simulink library "motion"  (Simulink 4.00)
undefined symbols (not defined in the file or in its folder): A6, Ac, Acd, ad, Aff, Aff0, Aff6, Ap, As, B6, Bc, Bcd, Bff, Bff0, Bff6, Bp, Bs, C6, Cc, Ccd, Cff, Cff0, Cff6, Cp, Cs, D6, Dc, dd, Ddd, Dff, Dff0, Dff6, Dp, Ds, jd, Ts, Tsettle
libraries: motion x5
(part 2 of 4)

== system motion/Feedforward Controllers/Feedforward ==
  In1 : Inport  Port=1
  4th order continuous : motion/Feedforward Controllers/4th order continuous  m1=20  m2=10  k1=10  k2=10  c=6e5  k12=500
  Out1 : Outport  Port=1
  wires:
  In1/1 -> 4th order continuous/1
  4th order continuous/1 -> Out1/1

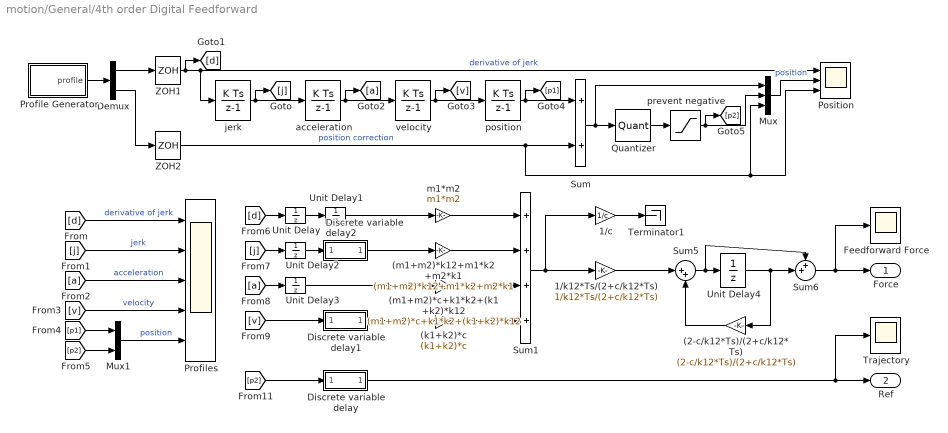
== system motion/General/4th order Digital Feedforward ==
  (2-c/k12*Ts)/(2+c/k12*Ts) : Gain  Orientation=left  Gain=(2-c/k12*Ts)/(2+c/k12*Ts)  Multiplication=Element-wise(K.*u)  SaturateOnIntegerOverflow=on
  (k1+k2)*c : Gain  Gain=(k1+k2)*c  Multiplication=Element-wise(K.*u)  SaturateOnIntegerOverflow=on
  (m1+m2)*c+k1*k2+(k1+k2)*k12 : Gain  Gain=(m1+m2)*c+k1*k2+(k1+k2)*k12  Multiplication=Element-wise(K.*u)  SaturateOnIntegerOverflow=on
  (m1+m2)*k12+m1*k2+m2*k1 : Gain  Gain=(m1+m2)*k12+m1*k2+m2*k1  Multiplication=Element-wise(K.*u)  SaturateOnIntegerOverflow=on
  1/c : Gain  Gain=1/c  Multiplication=Element-wise(K.*u)  SaturateOnIntegerOverflow=on
  1/k12*Ts/(2+c/k12*Ts) : Gain  Gain=1/k12*Ts/(2+c/k12*Ts)  Multiplication=Element-wise(K.*u)  SaturateOnIntegerOverflow=on
  Demux : Demux  Outputs=2  BusSelectionMode=off
  Discrete variable delay : Subsystem  mask{Ts=Ts, alpha=.5}
      mask prompts: Ts "Sample time"; alpha "Delay factor (between 0 and 1)"
      settings: RTWFcnNameOpts=Auto  RTWFileNameOpts=Auto
      mask Display: disp(sprintf('%3.1f*Ts',alpha))
  Discrete variable delay1 : Subsystem  mask{Ts=Ts, alpha=.5}
      mask prompts: Ts "Sample time"; alpha "Delay factor (between 0 and 1)"
      settings: RTWFcnNameOpts=Auto  RTWFileNameOpts=Auto
      mask Display: disp(sprintf('%3.1f*Ts',alpha))
  Discrete variable delay2 : Subsystem  mask{Ts=Ts, alpha=.5}
      mask prompts: Ts "Sample time"; alpha "Delay factor (between 0 and 1)"
      settings: RTWFcnNameOpts=Auto  RTWFileNameOpts=Auto
      mask Display: disp(sprintf('%3.1f*Ts',alpha))
  Feedforward Force : Scope
      settings: TimeRange=3  YMin=-150  YMax=200  SaveToWorkspace=off  SaveName=ScopeData  LimitDataPoints=on  MaxDataPoints=50000
  Mux : Mux  Inputs=3
  Mux1 : Mux  Inputs=2
  Position : Scope  NumInputPorts=3
      settings: TimeRange=3  YMin=-1000~-0.5~-0.0004  YMax=1000~1~0  SaveToWorkspace=off  SaveName=ScopeData2  LimitDataPoints=on  MaxDataPoints=50000
  Profile Generator : Subsystem  BlockChoice=dJerk with error correction
      link override dJerk with error correction: t0=t0  x=x  v=v  a=a  j=j  d=d  Ts=Ts  r=r  s=s
      settings: AttributesFormatString=%<BlockChoice>  TemplateBlock=motion/Profile Generators/Profile Generator  MemberBlocks=Acceleration,Derivative of Jerk,Jerk,dJerk with error correction  RTWFcnNameOpts=Auto  RTWFileNameOpts=Auto
  Profiles : Scope  NumInputPorts=5
      settings: TimeRange=3  YMin=-1000~-50~-5~-7.49453e-017~0  YMax=1000~50~5~1~1  SaveToWorkspace=off  SaveName=ScopeData4  LimitDataPoints=on  MaxDataPoints=50000
  Quantizer : Quantizer  QuantizationInterval=r  LinearizeAsGain=on
  Sum : Sum  Inputs=++  SaturateOnIntegerOverflow=on
  Sum1 : Sum  Inputs=++++  SaturateOnIntegerOverflow=on
  Sum5 : Sum  Inputs=|++  SaturateOnIntegerOverflow=on
  Sum6 : Sum  Inputs=++|  SaturateOnIntegerOverflow=on
  Terminator1 : Terminator
  Trajectory : Scope
      settings: TimeRange=3  YMin=0  YMax=1  SaveToWorkspace=off  SaveName=ScopeData7  LimitDataPoints=on  MaxDataPoints=50000
  Unit Delay{,1..4} (5 alike) : UnitDelay  X0=0  SampleTime=Ts
  ZOH1 : ZeroOrderHold  SampleTime=Ts
  ZOH2 : ZeroOrderHold  SampleTime=Ts
  acceleration : DiscreteIntegrator  IntegratorMethod=ForwardEuler  ExternalReset=none  InitialConditionSource=internal  InitialCondition=0  LimitOutput=off  UpperSaturationLimit=inf  LowerSaturationLimit=-inf  ShowSaturationPort=off  ShowStatePort=off  SampleTime=Ts
  jerk : DiscreteIntegrator  IntegratorMethod=ForwardEuler  ExternalReset=none  InitialConditionSource=internal  InitialCondition=0  LimitOutput=off  UpperSaturationLimit=inf  LowerSaturationLimit=-inf  ShowSaturationPort=off  ShowStatePort=off  SampleTime=Ts
  m1*m2 : Gain  Gain=m1*m2  Multiplication=Element-wise(K.*u)  SaturateOnIntegerOverflow=on
  position : DiscreteIntegrator  IntegratorMethod=ForwardEuler  ExternalReset=none  InitialConditionSource=internal  InitialCondition=0  LimitOutput=off  UpperSaturationLimit=inf  LowerSaturationLimit=-inf  ShowSaturationPort=off  ShowStatePort=off  SampleTime=Ts
  "prevent negative " : Saturate  UpperLimit=inf  LowerLimit=0  LinearizeAsGain=on
  velocity : DiscreteIntegrator  IntegratorMethod=ForwardEuler  ExternalReset=none  InitialConditionSource=internal  InitialCondition=0  LimitOutput=off  UpperSaturationLimit=inf  LowerSaturationLimit=-inf  ShowSaturationPort=off  ShowStatePort=off  SampleTime=Ts
  Force : Outport  Port=1
  Ref : Outport  Port=2
  wires:
  m1*m2/1 -> Sum1/1
  Profile Generator/1(profile) -> Demux/1
  (m1+m2)*k12+m1*k2+m2*k1/1 -> Sum1/2
  1/c/1 -> Terminator1/1
  Sum6/1 -> Force/1, Feedforward Force/1
  (2-c/k12*Ts)/(2+c/k12*Ts)/1 -> Sum5/2
  Unit Delay4/1 -> Sum6/2, (2-c/k12*Ts)/(2+c/k12*Ts)/1
  Sum5/1 -> Sum6/1, Unit Delay4/1
  1/k12*Ts/(2+c/k12*Ts)/1 -> Sum5/1
  Discrete variable delay2/1(Out1) -> (m1+m2)*k12+m1*k2+m2*k1/1
  Discrete variable delay1/1(Out1) -> (k1+k2)*c/1
  Unit Delay3/1 -> (m1+m2)*c+k1*k2+(k1+k2)*k12/1
  Unit Delay2/1 -> Discrete variable delay2/1(In1)
  Unit Delay1/1 -> m1*m2/1
  Unit Delay/1 -> Unit Delay1/1
  "prevent negative "/1 -> [p2], Mux/2
  Discrete variable delay/1(Out1) -> Ref/1, Trajectory/1
  [p2] -> Discrete variable delay/1(In1)
  Sum1/1 -> 1/k12*Ts/(2+c/k12*Ts)/1, 1/c/1
  (k1+k2)*c/1 -> Sum1/4
  (m1+m2)*c+k1*k2+(k1+k2)*k12/1 -> Sum1/3
  [v] -> Discrete variable delay1/1(In1)
  [a] -> Unit Delay3/1
  [j] -> Unit Delay2/1
  [d] -> Unit Delay/1
  Mux1/1 -> Profiles/5  "position"
  [v] -> Profiles/4  "velocity"
  [a] -> Profiles/3  "acceleration"
  [j] -> Profiles/2  "jerk"
  [d] -> Profiles/1  "derivative of jerk"
  [p2] -> Mux1/2
  [p1] -> Mux1/1
  ZOH2/1 -> Position/3, Mux/3, Sum/2  "position correction"
  position/1 -> [p1], Sum/1
  Mux/1 -> Position/2  "position"
  Sum/1 -> Mux/1, Quantizer/1
  Quantizer/1 -> "prevent negative "/1
  Demux/2 -> ZOH2/1
  ZOH1/1 -> [d], Position/1, jerk/1  "derivative of jerk"
  velocity/1 -> [v], position/1
  acceleration/1 -> [a], velocity/1
  jerk/1 -> [j], acceleration/1
  Demux/1 -> ZOH1/1

== system motion/General/open example ==
  note: Run makeplant

== system motion/General/open example1 ==
  note: Run makeplant

== system motion/General/open example2 ==
  note: Run makeplant

== system motion/General/run makeplant ==
  note: Run makeplant

== system motion/Motion Systems1/Motion System ==
  In1 : Inport  Port=1
  2nd order : StateSpace  A=As  B=Bs  C=Cs  D=Ds  X0=0  Realization=auto  AbsoluteTolerance=auto
  Out1 : Outport  Port=1
  wires:
  In1/1 -> 2nd order/1
  2nd order/1 -> Out1/1

== system motion/Motion Systems1/Parametrized 4th order ==
  In1 : Inport  Port=1
  4th order plant1 : StateSpace  A=Ap  B=Bp  C=Cp  D=Dp  X0=0  Realization=auto  AbsoluteTolerance=auto
  Out1 : Outport  Port=1
  wires:
  4th order plant1/1 -> Out1/1
  In1/1 -> 4th order plant1/1

== system motion/Profile Generators/Acceleration ==
  Sum : Sum  Inputs=4  SaturateOnIntegerOverflow=on
  t0 : Step  Time=t0  Before=0  After=ad(1)  SampleTime=0
  t1 : Step  Time=t0+t(1)  Before=0  After=-ad(1)  SampleTime=0
  t2 : Step  Time=t0+t(1)+t(2)  Before=0  After=-ad(1)  SampleTime=0
  t3 : Step  Time=t0+2*t(1)+t(2)  Before=0  After=ad(1)  SampleTime=0
  profile : Outport  Port=1
  wires:
  t0/1 -> Sum/1
  t1/1 -> Sum/2
  t2/1 -> Sum/3
  t3/1 -> Sum/4
  Sum/1 -> profile/1

== system motion/Profile Generators/Derivative of Jerk ==
  Sum : Sum  Inputs=16  SaturateOnIntegerOverflow=on
  t0 : Step  Time=t0  Before=0  After=dd(1)  SampleTime=0
  t1 : Step  Time=t0+t(1)  Before=0  After=-dd(1)  SampleTime=0
  t10 : Step  Time=t0+5*t(1)+3*t(2)+t(3)+t(4)  Before=0  After=dd(1)  SampleTime=0
  t11 : Step  Time=t0+6*t(1)+3*t(2)+t(3)+t(4)  Before=0  After=-dd(1)  SampleTime=0
  t12 : Step  Time=t0+6*t(1)+3*t(2)+2*t(3)+t(4)  Before=0  After=dd(1)  SampleTime=0
  t13 : Step  Time=t0+7*t(1)+3*t(2)+2*t(3)+t(4)  Before=0  After=-dd(1)  SampleTime=0
  t14 : Step  Time=t0+7*t(1)+4*t(2)+2*t(3)+t(4)  Before=0  After=-dd(1)  SampleTime=0
  t15 : Step  Time=t0+8*t(1)+4*t(2)+2*t(3)+t(4)  Before=0  After=dd(1)  SampleTime=0
  t2 : Step  Time=t0+t(1)+t(2)  Before=0  After=-dd(1)  SampleTime=0
  t3 : Step  Time=t0+2*t(1)+t(2)  Before=0  After=dd(1)  SampleTime=0
  t4 : Step  Time=t0+2*t(1)+t(2)+t(3)  Before=0  After=-dd(1)  SampleTime=0
  t5 : Step  Time=t0+3*t(1)+t(2)+t(3)  Before=0  After=dd(1)  SampleTime=0
  t6 : Step  Time=t0+3*t(1)+2*t(2)+t(3)  Before=0  After=dd(1)  SampleTime=0
  t7 : Step  Time=t0+4*t(1)+2*t(2)+t(3)  Before=0  After=-dd(1)  SampleTime=0
  t8 : Step  Time=t0+4*t(1)+2*t(2)+t(3)+t(4)  Before=0  After=-dd(1)  SampleTime=0
  t9 : Step  Time=t0+5*t(1)+2*t(2)+t(3)+t(4)  Before=0  After=dd(1)  SampleTime=0
  profile : Outport  Port=1
  wires:
  t0/1 -> Sum/1
  t1/1 -> Sum/2
  t2/1 -> Sum/3
  t3/1 -> Sum/4
  t4/1 -> Sum/5
  t5/1 -> Sum/6
  t6/1 -> Sum/7
  t7/1 -> Sum/8
  t8/1 -> Sum/9
  t9/1 -> Sum/10
  t10/1 -> Sum/11
  t11/1 -> Sum/12
  t12/1 -> Sum/13
  t13/1 -> Sum/14
  t14/1 -> Sum/15
  t15/1 -> Sum/16
  Sum/1 -> profile/1

== system motion/Profile Generators/Jerk ==
  Sum : Sum  Inputs=8  SaturateOnIntegerOverflow=on
  t0 : Step  Time=t0  Before=0  After=jd(1)  SampleTime=0
  t1 : Step  Time=t0+t(1)  Before=0  After=-jd(1)  SampleTime=0
  t2 : Step  Time=t0+t(1)+t(2)  Before=0  After=-jd(1)  SampleTime=0
  t3 : Step  Time=t0+2*t(1)+t(2)  Before=0  After=jd(1)  SampleTime=0
  t4 : Step  Time=t0+2*t(1)+t(2)+t(3)  Before=0  After=-jd(1)  SampleTime=0
  t5 : Step  Time=t0+3*t(1)+t(2)+t(3)  Before=0  After=jd(1)  SampleTime=0
  t6 : Step  Time=t0+3*t(1)+2*t(2)+t(3)  Before=0  After=jd(1)  SampleTime=0
  t7 : Step  Time=t0+4*t(1)+2*t(2)+t(3)  Before=0  After=-jd(1)  SampleTime=0
  profile : Outport  Port=1
  wires:
  Sum/1 -> profile/1
  t7/1 -> Sum/8
  t6/1 -> Sum/7
  t5/1 -> Sum/6
  t4/1 -> Sum/5
  t3/1 -> Sum/4
  t2/1 -> Sum/3
  t1/1 -> Sum/2
  t0/1 -> Sum/1

== system motion/Profile Generators/Profile Generator ==
  Acceleration : motion/Profile Generators/Acceleration  t0=.3  x=1  v=1  a=5  Ts=0
  profile : Outport  Port=1
  wires:
  Acceleration/1 -> profile/1

== system motion/Profile Generators/dJerk with error correction ==
  Clock : Clock
      settings: DisplayTime=off  Decimation=10
  Correction at start of trajectory : Lookup  InputValues="[ -1 t0 t0+abs(dd(3))*Ts  2*(t0+8*t(1)+4*t(2)+2*t(3)+t(4)) ]"  OutputValues=[ 0 0 [1 1]*dd(3)*r]
  Correction during entire trajectory : Lookup  InputValues="[ -1 t0  t0+8*t(1)+4*t(2)+2*t(3)+t(4)  2*(t0+8*t(1)+4*t(2)+2*t(3)+t(4)) ]"  OutputValues=[0 0 [1 1]*dd(2)*r]
  Mux : Mux  Inputs=2
  Sum : Sum  Inputs=16  SaturateOnIntegerOverflow=on
  Sum1 : Sum  Inputs=|++  SaturateOnIntegerOverflow=on
  t0 : Step  Time=t0  Before=0  After=dd(1)  SampleTime=0
  t1 : Step  Time=t0+t(1)  Before=0  After=-dd(1)  SampleTime=0
  t10 : Step  Time=t0+5*t(1)+3*t(2)+t(3)+t(4)  Before=0  After=dd(1)  SampleTime=0
  t11 : Step  Time=t0+6*t(1)+3*t(2)+t(3)+t(4)  Before=0  After=-dd(1)  SampleTime=0
  t12 : Step  Time=t0+6*t(1)+3*t(2)+2*t(3)+t(4)  Before=0  After=dd(1)  SampleTime=0
  t13 : Step  Time=t0+7*t(1)+3*t(2)+2*t(3)+t(4)  Before=0  After=-dd(1)  SampleTime=0
  t14 : Step  Time=t0+7*t(1)+4*t(2)+2*t(3)+t(4)  Before=0  After=-dd(1)  SampleTime=0
  t15 : Step  Time=t0+8*t(1)+4*t(2)+2*t(3)+t(4)  Before=0  After=dd(1)  SampleTime=0
  t2 : Step  Time=t0+t(1)+t(2)  Before=0  After=-dd(1)  SampleTime=0
  t3 : Step  Time=t0+2*t(1)+t(2)  Before=0  After=dd(1)  SampleTime=0
  t4 : Step  Time=t0+2*t(1)+t(2)+t(3)  Before=0  After=-dd(1)  SampleTime=0
  t5 : Step  Time=t0+3*t(1)+t(2)+t(3)  Before=0  After=dd(1)  SampleTime=0
  t6 : Step  Time=t0+3*t(1)+2*t(2)+t(3)  Before=0  After=dd(1)  SampleTime=0
  t7 : Step  Time=t0+4*t(1)+2*t(2)+t(3)  Before=0  After=-dd(1)  SampleTime=0
  t8 : Step  Time=t0+4*t(1)+2*t(2)+t(3)+t(4)  Before=0  After=-dd(1)  SampleTime=0
  t9 : Step  Time=t0+5*t(1)+2*t(2)+t(3)+t(4)  Before=0  After=dd(1)  SampleTime=0
  profile : Outport  Port=1
  wires:
  Sum/1 -> Mux/1
  Mux/1 -> profile/1
  t0/1 -> Sum/1
  t1/1 -> Sum/2
  t2/1 -> Sum/3
  t3/1 -> Sum/4
  t4/1 -> Sum/5
  t5/1 -> Sum/6
  t6/1 -> Sum/7
  t7/1 -> Sum/8
  t8/1 -> Sum/9
  t9/1 -> Sum/10
  t10/1 -> Sum/11
  t11/1 -> Sum/12
  t12/1 -> Sum/13
  t13/1 -> Sum/14
  t14/1 -> Sum/15
  t15/1 -> Sum/16
  Clock/1 -> Correction during entire trajectory/1, Correction at start of trajectory/1
  Correction at start of trajectory/1 -> Sum1/2
  Sum1/1 -> Mux/2
  Correction during entire trajectory/1 -> Sum1/1

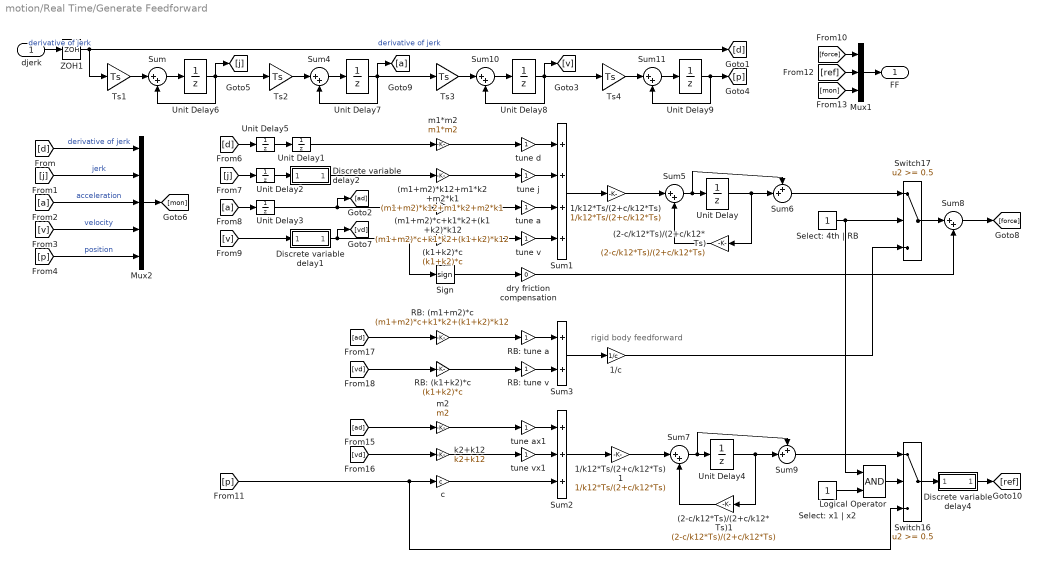
== system motion/Real Time/Generate Feedforward ==
  note: rigid body feedforward
  djerk : Inport  Port=1
  (2-c/k12*Ts)/(2+c/k12*Ts) : Gain  Orientation=left  Gain=(2-c/k12*Ts)/(2+c/k12*Ts)  Multiplication=Element-wise(K.*u)  SaturateOnIntegerOverflow=on
  (2-c/k12*Ts)/(2+c/k12*Ts)1 : Gain  Orientation=left  Gain=(2-c/k12*Ts)/(2+c/k12*Ts)  Multiplication=Element-wise(K.*u)  SaturateOnIntegerOverflow=on
  (k1+k2)*c : Gain  Gain=(k1+k2)*c  Multiplication=Element-wise(K.*u)  SaturateOnIntegerOverflow=on
  (m1+m2)*c+k1*k2+(k1+k2)*k12 : Gain  Gain=(m1+m2)*c+k1*k2+(k1+k2)*k12  Multiplication=Element-wise(K.*u)  SaturateOnIntegerOverflow=on
  (m1+m2)*k12+m1*k2+m2*k1 : Gain  Gain=(m1+m2)*k12+m1*k2+m2*k1  Multiplication=Element-wise(K.*u)  SaturateOnIntegerOverflow=on
  1/c : Gain  Gain=1/c  Multiplication=Element-wise(K.*u)  SaturateOnIntegerOverflow=on
  1/k12*Ts/(2+c/k12*Ts) : Gain  Gain=1/k12*Ts/(2+c/k12*Ts)  Multiplication=Element-wise(K.*u)  SaturateOnIntegerOverflow=on
  1/k12*Ts/(2+c/k12*Ts)1 : Gain  Gain=1/k12*Ts/(2+c/k12*Ts)  Multiplication=Element-wise(K.*u)  SaturateOnIntegerOverflow=on
  Discrete variable delay1 : Subsystem  mask{Ts=Ts, alpha=.5}
      mask prompts: Ts "Sample time"; alpha "Delay factor (between 0 and 1)"
      settings: RTWFcnNameOpts=Auto  RTWFileNameOpts=Auto
      mask Display: disp(sprintf('%3.1f*Ts',alpha))
  Discrete variable delay2 : Subsystem  mask{Ts=Ts, alpha=.5}
      mask prompts: Ts "Sample time"; alpha "Delay factor (between 0 and 1)"
      settings: RTWFcnNameOpts=Auto  RTWFileNameOpts=Auto
      mask Display: disp(sprintf('%3.1f*Ts',alpha))
  Discrete variable delay4 : Subsystem  mask{Ts=Ts, alpha=.5}
      mask prompts: Ts "Sample time"; alpha "Delay factor (between 0 and 1)"
      settings: RTWFcnNameOpts=Auto  RTWFileNameOpts=Auto
      mask Display: disp(sprintf('%3.1f*Ts',alpha))
  Logical Operator : Logic  Operator=AND  Inputs=2
  Mux1 : Mux  Inputs=3
  Mux2 : Mux  Inputs=5
  RB: (k1+k2)*c : Gain  Gain=(k1+k2)*c  Multiplication=Element-wise(K.*u)  SaturateOnIntegerOverflow=on
  RB: (m1+m2)*c : Gain  Gain=(m1+m2)*c+k1*k2+(k1+k2)*k12  Multiplication=Element-wise(K.*u)  SaturateOnIntegerOverflow=on
  RB: tune a : Gain  Gain=1  Multiplication=Element-wise(K.*u)  SaturateOnIntegerOverflow=on
  RB: tune v : Gain  Gain=1  Multiplication=Element-wise(K.*u)  SaturateOnIntegerOverflow=on
  Select: 4th | RB : Constant  Value=1
  Select: x1 | x2 : Constant  Value=1
  Sign : Signum
  Sum{,4..5,7..8,10..11} (7 alike) : Sum  Inputs=|++  SaturateOnIntegerOverflow=on
  Sum1 : Sum  Inputs=++++  SaturateOnIntegerOverflow=on
  Sum2 : Sum  Inputs=+++  SaturateOnIntegerOverflow=on
  Sum3 : Sum  Inputs=++  SaturateOnIntegerOverflow=on
  Sum6 : Sum  Inputs=++|  SaturateOnIntegerOverflow=on
  Sum9 : Sum  Inputs=++|  SaturateOnIntegerOverflow=on
  Switch16 : Switch  Threshold=0.5
  Switch17 : Switch  Threshold=0.5
  Ts{1..4} (4 alike) : Gain  Gain=Ts  Multiplication=Element-wise(K.*u)  SaturateOnIntegerOverflow=on
  Unit Delay{,1..9} (10 alike) : UnitDelay  X0=0  SampleTime=Ts
  ZOH1 : ZeroOrderHold  SampleTime=Ts
  c : Gain  Gain=c  Multiplication=Element-wise(K.*u)  SaturateOnIntegerOverflow=on
  dry friction compensation : Gain  Gain=0  Multiplication=Element-wise(K.*u)  SaturateOnIntegerOverflow=on
  k2+k12 : Gain  Gain=k2+k12  Multiplication=Element-wise(K.*u)  SaturateOnIntegerOverflow=on
  m1*m2 : Gain  Gain=m1*m2  Multiplication=Element-wise(K.*u)  SaturateOnIntegerOverflow=on
  m2 : Gain  Gain=m2  Multiplication=Element-wise(K.*u)  SaturateOnIntegerOverflow=on
  tune a : Gain  Gain=1  Multiplication=Element-wise(K.*u)  SaturateOnIntegerOverflow=on
  tune ax1 : Gain  Gain=1  Multiplication=Element-wise(K.*u)  SaturateOnIntegerOverflow=on
  tune d : Gain  Gain=1  Multiplication=Element-wise(K.*u)  SaturateOnIntegerOverflow=on
  tune j : Gain  Gain=1  Multiplication=Element-wise(K.*u)  SaturateOnIntegerOverflow=on
  tune v : Gain  Gain=1  Multiplication=Element-wise(K.*u)  SaturateOnIntegerOverflow=on
  tune vx1 : Gain  Gain=1  Multiplication=Element-wise(K.*u)  SaturateOnIntegerOverflow=on
  FF : Outport  Port=1
  wires:
  Sum11/1 -> Unit Delay9/1
  Ts4/1 -> Sum11/1
  Unit Delay9/1 -> [p], Sum11/2
  Sum10/1 -> Unit Delay8/1
  Ts3/1 -> Sum10/1
  Unit Delay8/1 -> Ts4/1, [v], Sum10/2
  Sum4/1 -> Unit Delay7/1
  Ts2/1 -> Sum4/1
  Unit Delay7/1 -> Ts3/1, [a], Sum4/2
  Sum/1 -> Unit Delay6/1
  Ts1/1 -> Sum/1
  Unit Delay6/1 -> Ts2/1, [j], Sum/2
  c/1 -> Sum2/3
  Select: 4th | RB/1 -> Logical Operator/1, Switch17/2
  Sum9/1 -> Switch16/1
  1/c/1 -> Switch17/3
  dry friction compensation/1 -> Sum8/2
  Logical Operator/1 -> Switch16/2
  Select: x1 | x2/1 -> Logical Operator/2
  Discrete variable delay4/1(Out1) -> [ref]
  Switch16/1 -> Discrete variable delay4/1(In1)
  Sum8/1 -> [force]
  Switch17/1 -> Sum8/1
  Sum6/1 -> Switch17/1
  Unit Delay4/1 -> Sum9/2, (2-c/k12*Ts)/(2+c/k12*Ts)1/1
  Sum7/1 -> Sum9/1, Unit Delay4/1
  1/k12*Ts/(2+c/k12*Ts)1/1 -> Sum7/1
  Sum2/1 -> 1/k12*Ts/(2+c/k12*Ts)1/1
  (2-c/k12*Ts)/(2+c/k12*Ts)1/1 -> Sum7/2
  [vd] -> k2+k12/1
  [ad] -> m2/1
  [p] -> c/1, Switch16/3
  m2/1 -> tune ax1/1
  tune ax1/1 -> Sum2/1
  k2+k12/1 -> tune vx1/1
  tune vx1/1 -> Sum2/2
  [ad] -> RB: (m1+m2)*c/1
  [vd] -> RB: (k1+k2)*c/1
  RB: (m1+m2)*c/1 -> RB: tune a/1
  RB: tune a/1 -> Sum3/1
  RB: (k1+k2)*c/1 -> RB: tune v/1
  RB: tune v/1 -> Sum3/2
  Sum3/1 -> 1/c/1
  [force] -> Mux1/1
  [ref] -> Mux1/2
  [mon] -> Mux1/3
  Mux1/1 -> FF/1
  Unit Delay3/1 -> [ad], (m1+m2)*c+k1*k2+(k1+k2)*k12/1
  Discrete variable delay2/1(Out1) -> (m1+m2)*k12+m1*k2+m2*k1/1
  Unit Delay1/1 -> m1*m2/1
  m1*m2/1 -> tune d/1
  tune d/1 -> Sum1/1
  (m1+m2)*k12+m1*k2+m2*k1/1 -> tune j/1
  tune j/1 -> Sum1/2
  (m1+m2)*c+k1*k2+(k1+k2)*k12/1 -> tune a/1
  tune a/1 -> Sum1/3
  (k1+k2)*c/1 -> tune v/1
  tune v/1 -> Sum1/4
  Unit Delay/1 -> Sum6/2, (2-c/k12*Ts)/(2+c/k12*Ts)/1
  Sum5/1 -> Sum6/1, Unit Delay/1
  1/k12*Ts/(2+c/k12*Ts)/1 -> Sum5/1
  Sum1/1 -> 1/k12*Ts/(2+c/k12*Ts)/1
  (2-c/k12*Ts)/(2+c/k12*Ts)/1 -> Sum5/2
  Sign/1 -> dry friction compensation/1
  djerk/1 -> ZOH1/1  "derivative of jerk"
  Unit Delay2/1 -> Discrete variable delay2/1(In1)
  Unit Delay5/1 -> Unit Delay1/1
  [v] -> Discrete variable delay1/1(In1)
  [a] -> Unit Delay3/1
  [j] -> Unit Delay2/1
  [d] -> Unit Delay5/1
  [v] -> Mux2/4  "velocity"
  [a] -> Mux2/3  "acceleration"
  [j] -> Mux2/2  "jerk"
  [d] -> Mux2/1  "derivative of jerk"
  [p] -> Mux2/5  "position"
  Mux2/1 -> [mon]
  ZOH1/1 -> Ts1/1, [d]  "derivative of jerk"
  Discrete variable delay1/1(Out1) -> [vd], (k1+k2)*c/1, Sign/1

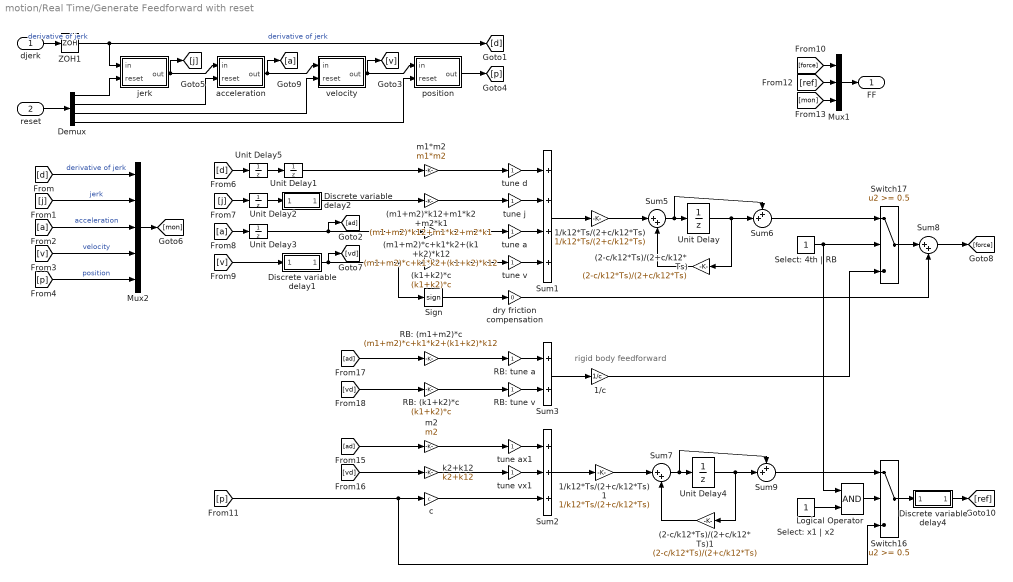
== system motion/Real Time/Generate Feedforward with reset ==
  note: rigid body feedforward
  djerk : Inport  Port=1
  reset : Inport  Port=2
  (2-c/k12*Ts)/(2+c/k12*Ts) : Gain  Orientation=left  Gain=(2-c/k12*Ts)/(2+c/k12*Ts)  Multiplication=Element-wise(K.*u)  SaturateOnIntegerOverflow=on
  (2-c/k12*Ts)/(2+c/k12*Ts)1 : Gain  Orientation=left  Gain=(2-c/k12*Ts)/(2+c/k12*Ts)  Multiplication=Element-wise(K.*u)  SaturateOnIntegerOverflow=on
  (k1+k2)*c : Gain  Gain=(k1+k2)*c  Multiplication=Element-wise(K.*u)  SaturateOnIntegerOverflow=on
  (m1+m2)*c+k1*k2+(k1+k2)*k12 : Gain  Gain=(m1+m2)*c+k1*k2+(k1+k2)*k12  Multiplication=Element-wise(K.*u)  SaturateOnIntegerOverflow=on
  (m1+m2)*k12+m1*k2+m2*k1 : Gain  Gain=(m1+m2)*k12+m1*k2+m2*k1  Multiplication=Element-wise(K.*u)  SaturateOnIntegerOverflow=on
  1/c : Gain  Gain=1/c  Multiplication=Element-wise(K.*u)  SaturateOnIntegerOverflow=on
  1/k12*Ts/(2+c/k12*Ts) : Gain  Gain=1/k12*Ts/(2+c/k12*Ts)  Multiplication=Element-wise(K.*u)  SaturateOnIntegerOverflow=on
  1/k12*Ts/(2+c/k12*Ts)1 : Gain  Gain=1/k12*Ts/(2+c/k12*Ts)  Multiplication=Element-wise(K.*u)  SaturateOnIntegerOverflow=on
  Demux : Demux  Outputs=4  BusSelectionMode=off
  Discrete variable delay1 : Subsystem  mask{Ts=Ts, alpha=.5}
      mask prompts: Ts "Sample time"; alpha "Delay factor (between 0 and 1)"
      settings: RTWFcnNameOpts=Auto  RTWFileNameOpts=Auto
      mask Display: disp(sprintf('%3.1f*Ts',alpha))
  Discrete variable delay2 : Subsystem  mask{Ts=Ts, alpha=.5}
      mask prompts: Ts "Sample time"; alpha "Delay factor (between 0 and 1)"
      settings: RTWFcnNameOpts=Auto  RTWFileNameOpts=Auto
      mask Display: disp(sprintf('%3.1f*Ts',alpha))
  Discrete variable delay4 : Subsystem  mask{Ts=Ts, alpha=.5}
      mask prompts: Ts "Sample time"; alpha "Delay factor (between 0 and 1)"
      settings: RTWFcnNameOpts=Auto  RTWFileNameOpts=Auto
      mask Display: disp(sprintf('%3.1f*Ts',alpha))
  Logical Operator : Logic  Operator=AND  Inputs=2
  Mux1 : Mux  Inputs=3
  Mux2 : Mux  Inputs=5
  RB: (k1+k2)*c : Gain  Gain=(k1+k2)*c  Multiplication=Element-wise(K.*u)  SaturateOnIntegerOverflow=on
  RB: (m1+m2)*c : Gain  Gain=(m1+m2)*c+k1*k2+(k1+k2)*k12  Multiplication=Element-wise(K.*u)  SaturateOnIntegerOverflow=on
  RB: tune a : Gain  Gain=1  Multiplication=Element-wise(K.*u)  SaturateOnIntegerOverflow=on
  RB: tune v : Gain  Gain=1  Multiplication=Element-wise(K.*u)  SaturateOnIntegerOverflow=on
  Select: 4th | RB : Constant  Value=1
  Select: x1 | x2 : Constant  Value=1
  Sign : Signum
  Sum1 : Sum  Inputs=++++  SaturateOnIntegerOverflow=on
  Sum2 : Sum  Inputs=+++  SaturateOnIntegerOverflow=on
  Sum3 : Sum  Inputs=++  SaturateOnIntegerOverflow=on
  Sum5 : Sum  Inputs=|++  SaturateOnIntegerOverflow=on
  Sum6 : Sum  Inputs=++|  SaturateOnIntegerOverflow=on
  Sum7 : Sum  Inputs=|++  SaturateOnIntegerOverflow=on
  Sum8 : Sum  Inputs=|++  SaturateOnIntegerOverflow=on
  Sum9 : Sum  Inputs=++|  SaturateOnIntegerOverflow=on
  Switch16 : Switch  Threshold=0.5
  Switch17 : Switch  Threshold=0.5
  Unit Delay{,1..5} (6 alike) : UnitDelay  X0=0  SampleTime=Ts
  ZOH1 : ZeroOrderHold  SampleTime=Ts
  acceleration : Subsystem
      settings: RTWFcnNameOpts=Auto  RTWFileNameOpts=Auto
  c : Gain  Gain=c  Multiplication=Element-wise(K.*u)  SaturateOnIntegerOverflow=on
  dry friction compensation : Gain  Gain=0  Multiplication=Element-wise(K.*u)  SaturateOnIntegerOverflow=on
  jerk : Subsystem
      settings: RTWFcnNameOpts=Auto  RTWFileNameOpts=Auto
  k2+k12 : Gain  Gain=k2+k12  Multiplication=Element-wise(K.*u)  SaturateOnIntegerOverflow=on
  m1*m2 : Gain  Gain=m1*m2  Multiplication=Element-wise(K.*u)  SaturateOnIntegerOverflow=on
  m2 : Gain  Gain=m2  Multiplication=Element-wise(K.*u)  SaturateOnIntegerOverflow=on
  position : Subsystem
      settings: RTWFcnNameOpts=Auto  RTWFileNameOpts=Auto
  tune a : Gain  Gain=1  Multiplication=Element-wise(K.*u)  SaturateOnIntegerOverflow=on
  tune ax1 : Gain  Gain=1  Multiplication=Element-wise(K.*u)  SaturateOnIntegerOverflow=on
  tune d : Gain  Gain=1  Multiplication=Element-wise(K.*u)  SaturateOnIntegerOverflow=on
  tune j : Gain  Gain=1  Multiplication=Element-wise(K.*u)  SaturateOnIntegerOverflow=on
  tune v : Gain  Gain=1  Multiplication=Element-wise(K.*u)  SaturateOnIntegerOverflow=on
  tune vx1 : Gain  Gain=1  Multiplication=Element-wise(K.*u)  SaturateOnIntegerOverflow=on
  velocity : Subsystem
      settings: RTWFcnNameOpts=Auto  RTWFileNameOpts=Auto
  FF : Outport  Port=1
  wires:
  position/1(out) -> [p]
  Discrete variable delay1/1(Out1) -> Sign/1, (k1+k2)*c/1, [vd]
  Demux/4 -> position/2(reset)
  velocity/1(out) -> position/1(in), [v]
  Demux/3 -> velocity/2(reset)
  Demux/2 -> acceleration/2(reset)
  Demux/1 -> jerk/2(reset)
  jerk/1(out) -> acceleration/1(in), [j]
  acceleration/1(out) -> velocity/1(in), [a]
  ZOH1/1 -> [d], jerk/1(in)  "derivative of jerk"
  reset/1 -> Demux/1
  Mux2/1 -> [mon]
  [p] -> Mux2/5  "position"
  [d] -> Mux2/1  "derivative of jerk"
  [j] -> Mux2/2  "jerk"
  [a] -> Mux2/3  "acceleration"
  [v] -> Mux2/4  "velocity"
  [d] -> Unit Delay5/1
  [j] -> Unit Delay2/1
  [a] -> Unit Delay3/1
  [v] -> Discrete variable delay1/1(In1)
  Unit Delay5/1 -> Unit Delay1/1
  Unit Delay2/1 -> Discrete variable delay2/1(In1)
  djerk/1 -> ZOH1/1  "derivative of jerk"
  Sign/1 -> dry friction compensation/1
  (2-c/k12*Ts)/(2+c/k12*Ts)/1 -> Sum5/2
  Sum1/1 -> 1/k12*Ts/(2+c/k12*Ts)/1
  1/k12*Ts/(2+c/k12*Ts)/1 -> Sum5/1
  Sum5/1 -> Unit Delay/1, Sum6/1
  Unit Delay/1 -> (2-c/k12*Ts)/(2+c/k12*Ts)/1, Sum6/2
  tune v/1 -> Sum1/4
  (k1+k2)*c/1 -> tune v/1
  tune a/1 -> Sum1/3
  (m1+m2)*c+k1*k2+(k1+k2)*k12/1 -> tune a/1
  tune j/1 -> Sum1/2
  (m1+m2)*k12+m1*k2+m2*k1/1 -> tune j/1
  tune d/1 -> Sum1/1
  m1*m2/1 -> tune d/1
  Unit Delay1/1 -> m1*m2/1
  Discrete variable delay2/1(Out1) -> (m1+m2)*k12+m1*k2+m2*k1/1
  Unit Delay3/1 -> (m1+m2)*c+k1*k2+(k1+k2)*k12/1, [ad]
  Mux1/1 -> FF/1
  [mon] -> Mux1/3
  [ref] -> Mux1/2
  [force] -> Mux1/1
  Sum3/1 -> 1/c/1
  RB: tune v/1 -> Sum3/2
  RB: (k1+k2)*c/1 -> RB: tune v/1
  RB: tune a/1 -> Sum3/1
  RB: (m1+m2)*c/1 -> RB: tune a/1
  [vd] -> RB: (k1+k2)*c/1
  [ad] -> RB: (m1+m2)*c/1
  tune vx1/1 -> Sum2/2
  k2+k12/1 -> tune vx1/1
  tune ax1/1 -> Sum2/1
  m2/1 -> tune ax1/1
  [p] -> Switch16/3, c/1
  [ad] -> m2/1
  [vd] -> k2+k12/1
  (2-c/k12*Ts)/(2+c/k12*Ts)1/1 -> Sum7/2
  Sum2/1 -> 1/k12*Ts/(2+c/k12*Ts)1/1
  1/k12*Ts/(2+c/k12*Ts)1/1 -> Sum7/1
  Sum7/1 -> Unit Delay4/1, Sum9/1
  Unit Delay4/1 -> (2-c/k12*Ts)/(2+c/k12*Ts)1/1, Sum9/2
  Sum6/1 -> Switch17/1
  Switch17/1 -> Sum8/1
  Sum8/1 -> [force]
  Switch16/1 -> Discrete variable delay4/1(In1)
  Discrete variable delay4/1(Out1) -> [ref]
  Select: x1 | x2/1 -> Logical Operator/2
  Logical Operator/1 -> Switch16/2
  dry friction compensation/1 -> Sum8/2
  1/c/1 -> Switch17/3
  Sum9/1 -> Switch16/1
  Select: 4th | RB/1 -> Switch17/2, Logical Operator/1
  c/1 -> Sum2/3

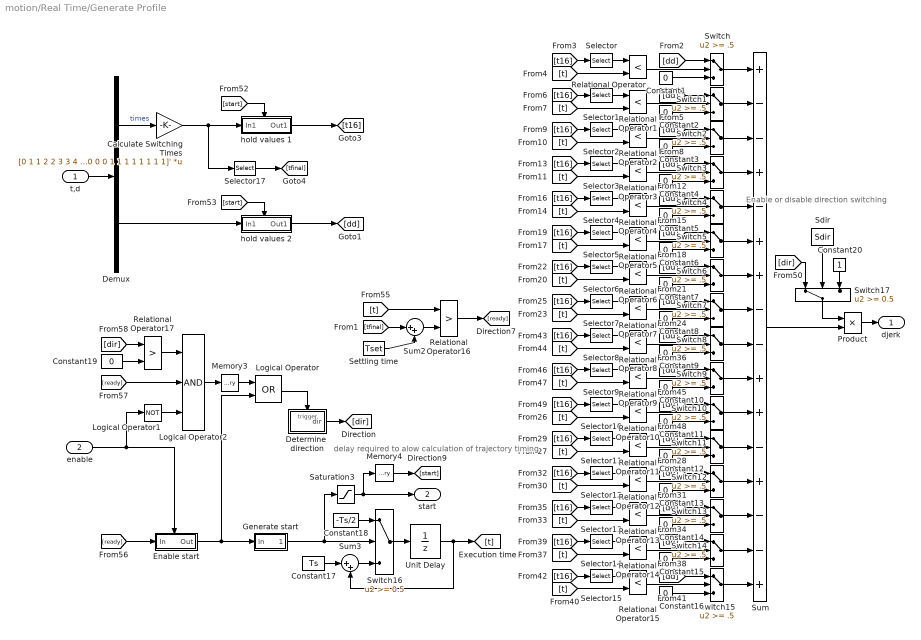
== system motion/Real Time/Generate Profile ==
  note: delay required to alow
      | calculation of trajectory timing
  note: Enable or disable
      | direction switching
  t,d : Inport  Port=1
  enable : Inport  Port=2
  Calculate Switching Times : Gain  Gain="[0 1 1 2 2 3 3 4 4 5 5 6 6 7 7 8 ; 0 0 1 1 1 1 2 2 2 2 3 3 3 3 4 4 ; 0 0 0 0 1 1 1 1 1 1 1 1 2 2 2 2 ;  0 0 0 0 0 0 0 0 1 1 1 1 1 1 1 1]'"  Multiplication=Matrix(K*u)  SaturateOnIntegerOverflow=on
  Constant{1..16,19} (17 alike) : Constant  Value=0
  Constant17 : Constant  Value=Ts
  Constant18 : Constant  Value=-Ts/2
  Constant20 : Constant  Orientation=down  Value=1
  Demux : Demux  Outputs=[4,1]  BusSelectionMode=off
  Determine  direction : Subsystem  TreatAsAtomicUnit=on
      settings: RTWFcnNameOpts=Auto  RTWFileNameOpts=Auto
  Enable start : Subsystem  TreatAsAtomicUnit=on
      settings: RTWFcnNameOpts=Auto  RTWFileNameOpts=Auto
  Generate start : Subsystem
      settings: RTWFcnNameOpts=Auto  RTWFileNameOpts=Auto
  Logical Operator : Logic  Operator=OR  Inputs=2
  Logical Operator1 : Logic  Operator=NOT  Inputs=2
  Logical Operator2 : Logic  Operator=AND  Inputs=3
  Memory3 : Memory  X0=0  InheritSampleTime=off
  Memory4 : Memory  X0=0  InheritSampleTime=off
  Product : Product  Inputs=2  Multiplication=Element-wise(.*)  SaturateOnIntegerOverflow=on
  Relational Operator{,1..15} (16 alike) : RelationalOperator  Operator=<
  Relational Operator16 : RelationalOperator  Operator=>
  Relational Operator17 : RelationalOperator  Operator=>
  Saturation3 : Saturate  UpperLimit=1  LowerLimit=0  LinearizeAsGain=on
  Sdir : Constant  Orientation=down  Value=Sdir
  Selector : Selector  InputType=Vector  ElementSrc=Internal  Elements=1  RowSrc=Internal  Rows=1  ColumnSrc=Internal  Columns=1  InputPortWidth=16
  Selector1 : Selector  InputType=Vector  ElementSrc=Internal  Elements=2  RowSrc=Internal  Rows=1  ColumnSrc=Internal  Columns=1  InputPortWidth=16
  Selector10 : Selector  InputType=Vector  ElementSrc=Internal  Elements=11  RowSrc=Internal  Rows=1  ColumnSrc=Internal  Columns=1  InputPortWidth=16
  Selector11 : Selector  InputType=Vector  ElementSrc=Internal  Elements=12  RowSrc=Internal  Rows=1  ColumnSrc=Internal  Columns=1  InputPortWidth=16
  Selector12 : Selector  InputType=Vector  ElementSrc=Internal  Elements=13  RowSrc=Internal  Rows=1  ColumnSrc=Internal  Columns=1  InputPortWidth=16
  Selector13 : Selector  InputType=Vector  ElementSrc=Internal  Elements=14  RowSrc=Internal  Rows=1  ColumnSrc=Internal  Columns=1  InputPortWidth=16
  Selector14 : Selector  InputType=Vector  ElementSrc=Internal  Elements=15  RowSrc=Internal  Rows=1  ColumnSrc=Internal  Columns=1  InputPortWidth=16
  Selector15 : Selector  InputType=Vector  ElementSrc=Internal  Elements=16  RowSrc=Internal  Rows=1  ColumnSrc=Internal  Columns=1  InputPortWidth=16
  Selector17 : Selector  InputType=Vector  ElementSrc=Internal  Elements=16  RowSrc=Internal  Rows=1  ColumnSrc=Internal  Columns=1  InputPortWidth=16
  Selector2 : Selector  InputType=Vector  ElementSrc=Internal  Elements=3  RowSrc=Internal  Rows=1  ColumnSrc=Internal  Columns=1  InputPortWidth=16
  Selector3 : Selector  InputType=Vector  ElementSrc=Internal  Elements=4  RowSrc=Internal  Rows=1  ColumnSrc=Internal  Columns=1  InputPortWidth=16
  Selector4 : Selector  InputType=Vector  ElementSrc=Internal  Elements=5  RowSrc=Internal  Rows=1  ColumnSrc=Internal  Columns=1  InputPortWidth=16
  Selector5 : Selector  InputType=Vector  ElementSrc=Internal  Elements=6  RowSrc=Internal  Rows=1  ColumnSrc=Internal  Columns=1  InputPortWidth=16
  Selector6 : Selector  InputType=Vector  ElementSrc=Internal  Elements=7  RowSrc=Internal  Rows=1  ColumnSrc=Internal  Columns=1  InputPortWidth=16
  Selector7 : Selector  InputType=Vector  ElementSrc=Internal  Elements=8  RowSrc=Internal  Rows=1  ColumnSrc=Internal  Columns=1  InputPortWidth=16
  Selector8 : Selector  InputType=Vector  ElementSrc=Internal  Elements=9  RowSrc=Internal  Rows=1  ColumnSrc=Internal  Columns=1  InputPortWidth=16
  Selector9 : Selector  InputType=Vector  ElementSrc=Internal  Elements=10  RowSrc=Internal  Rows=1  ColumnSrc=Internal  Columns=1  InputPortWidth=16
  Settling time : Constant  Value=Tset
  Sum : Sum  Inputs=+--+-++--++-+--+  SaturateOnIntegerOverflow=on
  Sum2 : Sum  Inputs=|++  SaturateOnIntegerOverflow=on
  Sum3 : Sum  Inputs=|++  SaturateOnIntegerOverflow=on
  Switch{,1..15} (16 alike) : Switch  Threshold=.5
  Switch16 : Switch  Threshold=0.5
  Switch17 : Switch  Orientation=down  Threshold=0.5
  Unit Delay : UnitDelay  X0=Tset-Ts/2  SampleTime=Ts
  hold values 1 : Subsystem  TreatAsAtomicUnit=on
      settings: RTWFcnNameOpts=Auto  RTWFileNameOpts=Auto
  hold values 2 : Subsystem  TreatAsAtomicUnit=on
      settings: RTWFcnNameOpts=Auto  RTWFileNameOpts=Auto
  djerk : Outport  Port=1
  start : Outport  Port=2
  wires:
  [tfinal] -> Sum2/1
  Relational Operator8/1 -> Switch8/2
  Saturation3/1 -> start/1, Memory4/1
  [start] -> hold values 2/Trigger
  [start] -> hold values 1/Trigger
  Memory4/1 -> [start]
  Relational Operator16/1 -> [ready]
  Sum2/1 -> Relational Operator16/2
  [t] -> Relational Operator16/1
  Settling time/1 -> Sum2/2
  Enable start/1(Out) -> Logical Operator/2, Generate start/1(In)
  Logical Operator2/1 -> Memory3/1
  Logical Operator1/1 -> Logical Operator2/3
  [dir] -> Relational Operator17/1
  Constant19/1 -> Relational Operator17/2
  [ready] -> Logical Operator2/2
  Relational Operator17/1 -> Logical Operator2/1
  Memory3/1 -> Logical Operator/1
  Determine  direction/1(dir) -> [dir]
  enable/1 -> Logical Operator1/1, Enable start/Enable
  [ready] -> Enable start/1(In)
  hold values 1/1(Out1) -> [t16]
  hold values 2/1(Out1) -> [dd]
  Demux/2 -> hold values 2/1(In1)
  Selector17/1 -> [tfinal]
  Calculate Switching Times/1 -> Selector17/1, hold values 1/1(In1)
  Demux/1 -> Calculate Switching Times/1  "times"
  t,d/1 -> Demux/1
  Relational Operator13/1 -> Switch13/2
  Relational Operator9/1 -> Switch9/2
  Relational Operator7/1 -> Switch7/2
  Relational Operator5/1 -> Switch5/2
  Relational Operator3/1 -> Switch3/2
  Relational Operator1/1 -> Switch1/2
  Relational Operator15/1 -> Switch15/2
  Constant16/1 -> Switch15/3
  [dd] -> Switch15/1
  Relational Operator11/1 -> Switch11/2
  Switch14/1 -> Sum/15
  Switch13/1 -> Sum/14
  Switch12/1 -> Sum/13
  Switch11/1 -> Sum/12
  Switch10/1 -> Sum/11
  Switch9/1 -> Sum/10
  Switch8/1 -> Sum/9
  Switch7/1 -> Sum/8
  Switch6/1 -> Sum/7
  Switch5/1 -> Sum/6
  Switch4/1 -> Sum/5
  Switch3/1 -> Sum/4
  Switch2/1 -> Sum/3
  Switch1/1 -> Sum/2
  Switch/1 -> Sum/1
  Relational Operator14/1 -> Switch14/2
  Constant15/1 -> Switch14/3
  [dd] -> Switch14/1
  Constant14/1 -> Switch13/3
  [dd] -> Switch13/1
  Relational Operator12/1 -> Switch12/2
  Constant13/1 -> Switch12/3
  [dd] -> Switch12/1
  Constant12/1 -> Switch11/3
  [dd] -> Switch11/1
  Relational Operator10/1 -> Switch10/2
  Constant11/1 -> Switch10/3
  [dd] -> Switch10/1
  Constant10/1 -> Switch9/3
  [dd] -> Switch9/1
  Constant9/1 -> Switch8/3
  [dd] -> Switch8/1
  Constant8/1 -> Switch7/3
  [dd] -> Switch7/1
  Relational Operator6/1 -> Switch6/2
  Constant7/1 -> Switch6/3
  [dd] -> Switch6/1
  Constant6/1 -> Switch5/3
  [dd] -> Switch5/1
  Relational Operator4/1 -> Switch4/2
  Constant5/1 -> Switch4/3
  [dd] -> Switch4/1
  Constant4/1 -> Switch3/3
  [dd] -> Switch3/1
  Relational Operator2/1 -> Switch2/2
  Constant3/1 -> Switch2/3
  [dd] -> Switch2/1
  Constant2/1 -> Switch1/3
  [dd] -> Switch1/1
  Relational Operator/1 -> Switch/2
  Constant1/1 -> Switch/3
  [dd] -> Switch/1
  Switch15/1 -> Sum/16
  [t] -> Relational Operator15/2
  Selector15/1 -> Relational Operator15/1
  [t16] -> Selector15/1
  [t] -> Relational Operator14/2
  Selector14/1 -> Relational Operator14/1
  [t16] -> Selector14/1
  [t] -> Relational Operator13/2
  Selector13/1 -> Relational Operator13/1
  [t16] -> Selector13/1
  [t] -> Relational Operator12/2
  Selector12/1 -> Relational Operator12/1
  [t16] -> Selector12/1
  [t] -> Relational Operator11/2
  Selector11/1 -> Relational Operator11/1
  [t16] -> Selector11/1
  [t] -> Relational Operator10/2
  Selector10/1 -> Relational Operator10/1
  [t16] -> Selector10/1
  [t] -> Relational Operator9/2
  Selector9/1 -> Relational Operator9/1
  [t16] -> Selector9/1
  [t] -> Relational Operator8/2
  Selector8/1 -> Relational Operator8/1
  [t16] -> Selector8/1
  [t] -> Relational Operator7/2
  Selector7/1 -> Relational Operator7/1
  [t16] -> Selector7/1
  [t] -> Relational Operator6/2
  Selector6/1 -> Relational Operator6/1
  [t16] -> Selector6/1
  [t] -> Relational Operator5/2
  Selector5/1 -> Relational Operator5/1
  [t16] -> Selector5/1
  [t] -> Relational Operator4/2
  Selector4/1 -> Relational Operator4/1
  [t16] -> Selector4/1
  [t] -> Relational Operator3/2
  Selector3/1 -> Relational Operator3/1
  [t16] -> Selector3/1
  [t] -> Relational Operator2/2
  Selector2/1 -> Relational Operator2/1
  [t16] -> Selector2/1
  [t] -> Relational Operator1/2
  Selector1/1 -> Relational Operator1/1
  [t16] -> Selector1/1
  [t] -> Relational Operator/2
  Selector/1 -> Relational Operator/1
  [t16] -> Selector/1
  Generate start/1(Out) -> Saturation3/1, Switch16/2
  Constant17/1 -> Sum3/1
  Unit Delay/1 -> Sum3/2, [t]
  Switch16/1 -> Unit Delay/1
  Sum3/1 -> Switch16/3
  Constant18/1 -> Switch16/1
  Product/1 -> djerk/1
  Logical Operator/1 -> Determine  direction/Trigger
  Sdir/1 -> Switch17/2
  Constant20/1 -> Switch17/3
  Sum/1 -> Product/2
  [dir] -> Switch17/1
  Switch17/1 -> Product/1

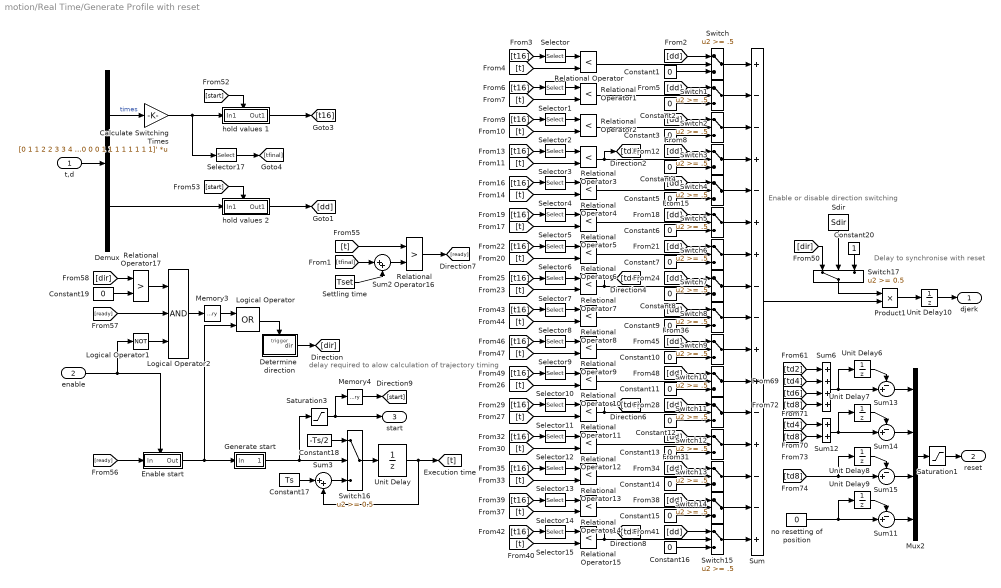
== system motion/Real Time/Generate Profile with reset ==
  note: delay required to alow
      | calculation of trajectory timing
  note: Enable or disable
      | direction switching
  note: Delay to
      | synchronise
      | with reset
  t,d : Inport  Port=1
  enable : Inport  Port=2
  Calculate Switching Times : Gain  Gain="[0 1 1 2 2 3 3 4 4 5 5 6 6 7 7 8 ; 0 0 1 1 1 1 2 2 2 2 3 3 3 3 4 4 ; 0 0 0 0 1 1 1 1 1 1 1 1 2 2 2 2 ;  0 0 0 0 0 0 0 0 1 1 1 1 1 1 1 1]'"  Multiplication=Matrix(K*u)  SaturateOnIntegerOverflow=on
  Constant{1..16,19} (17 alike) : Constant  Value=0
  Constant17 : Constant  Value=Ts
  Constant18 : Constant  Value=-Ts/2
  Constant20 : Constant  Orientation=down  Value=1
  Demux : Demux  Outputs=[4,1]  BusSelectionMode=off
  Determine  direction : Subsystem  TreatAsAtomicUnit=on
      settings: RTWFcnNameOpts=Auto  RTWFileNameOpts=Auto
  Enable start : Subsystem  TreatAsAtomicUnit=on
      settings: RTWFcnNameOpts=Auto  RTWFileNameOpts=Auto
  Generate start : Subsystem
      settings: RTWFcnNameOpts=Auto  RTWFileNameOpts=Auto
  Logical Operator : Logic  Operator=OR  Inputs=2
  Logical Operator1 : Logic  Operator=NOT  Inputs=2
  Logical Operator2 : Logic  Operator=AND  Inputs=3
  Memory3 : Memory  X0=0  InheritSampleTime=off
  Memory4 : Memory  X0=0  InheritSampleTime=off
  Mux2 : Mux  Inputs=4
  Product1 : Product  Inputs=2  Multiplication=Element-wise(.*)  SaturateOnIntegerOverflow=on
  Relational Operator{,1..15} (16 alike) : RelationalOperator  Operator=<
  Relational Operator16 : RelationalOperator  Operator=>
  Relational Operator17 : RelationalOperator  Operator=>
  Saturation1 : Saturate  UpperLimit=1  LowerLimit=0  LinearizeAsGain=on
  Saturation3 : Saturate  UpperLimit=1  LowerLimit=0  LinearizeAsGain=on
  Sdir : Constant  Orientation=down  Value=Sdir
  Selector : Selector  InputType=Vector  ElementSrc=Internal  Elements=1  RowSrc=Internal  Rows=1  ColumnSrc=Internal  Columns=1  InputPortWidth=16
  Selector1 : Selector  InputType=Vector  ElementSrc=Internal  Elements=2  RowSrc=Internal  Rows=1  ColumnSrc=Internal  Columns=1  InputPortWidth=16
  Selector10 : Selector  InputType=Vector  ElementSrc=Internal  Elements=11  RowSrc=Internal  Rows=1  ColumnSrc=Internal  Columns=1  InputPortWidth=16
  Selector11 : Selector  InputType=Vector  ElementSrc=Internal  Elements=12  RowSrc=Internal  Rows=1  ColumnSrc=Internal  Columns=1  InputPortWidth=16
  Selector12 : Selector  InputType=Vector  ElementSrc=Internal  Elements=13  RowSrc=Internal  Rows=1  ColumnSrc=Internal  Columns=1  InputPortWidth=16
  Selector13 : Selector  InputType=Vector  ElementSrc=Internal  Elements=14  RowSrc=Internal  Rows=1  ColumnSrc=Internal  Columns=1  InputPortWidth=16
  Selector14 : Selector  InputType=Vector  ElementSrc=Internal  Elements=15  RowSrc=Internal  Rows=1  ColumnSrc=Internal  Columns=1  InputPortWidth=16
  Selector15 : Selector  InputType=Vector  ElementSrc=Internal  Elements=16  RowSrc=Internal  Rows=1  ColumnSrc=Internal  Columns=1  InputPortWidth=16
  Selector17 : Selector  InputType=Vector  ElementSrc=Internal  Elements=16  RowSrc=Internal  Rows=1  ColumnSrc=Internal  Columns=1  InputPortWidth=16
  Selector2 : Selector  InputType=Vector  ElementSrc=Internal  Elements=3  RowSrc=Internal  Rows=1  ColumnSrc=Internal  Columns=1  InputPortWidth=16
  Selector3 : Selector  InputType=Vector  ElementSrc=Internal  Elements=4  RowSrc=Internal  Rows=1  ColumnSrc=Internal  Columns=1  InputPortWidth=16
  Selector4 : Selector  InputType=Vector  ElementSrc=Internal  Elements=5  RowSrc=Internal  Rows=1  ColumnSrc=Internal  Columns=1  InputPortWidth=16
  Selector5 : Selector  InputType=Vector  ElementSrc=Internal  Elements=6  RowSrc=Internal  Rows=1  ColumnSrc=Internal  Columns=1  InputPortWidth=16
  Selector6 : Selector  InputType=Vector  ElementSrc=Internal  Elements=7  RowSrc=Internal  Rows=1  ColumnSrc=Internal  Columns=1  InputPortWidth=16
  Selector7 : Selector  InputType=Vector  ElementSrc=Internal  Elements=8  RowSrc=Internal  Rows=1  ColumnSrc=Internal  Columns=1  InputPortWidth=16
  Selector8 : Selector  InputType=Vector  ElementSrc=Internal  Elements=9  RowSrc=Internal  Rows=1  ColumnSrc=Internal  Columns=1  InputPortWidth=16
  Selector9 : Selector  InputType=Vector  ElementSrc=Internal  Elements=10  RowSrc=Internal  Rows=1  ColumnSrc=Internal  Columns=1  InputPortWidth=16
  Settling time : Constant  Value=Tset
  Sum : Sum  Inputs=+--+-++--++-+--+  SaturateOnIntegerOverflow=on
  Sum{11,13..15} (4 alike) : Sum  Inputs=-+|  SaturateOnIntegerOverflow=on
  Sum12 : Sum  Inputs=++  SaturateOnIntegerOverflow=on
  Sum2 : Sum  Inputs=|++  SaturateOnIntegerOverflow=on
  Sum3 : Sum  Inputs=|++  SaturateOnIntegerOverflow=on
  Sum6 : Sum  Inputs=++++  SaturateOnIntegerOverflow=on
  Switch{,1..15} (16 alike) : Switch  Threshold=.5
  Switch16 : Switch  Threshold=0.5
  Switch17 : Switch  Orientation=down  Threshold=0.5
  Unit Delay : UnitDelay  X0=Tset-Ts/2  SampleTime=Ts
  Unit Delay{6..10} (5 alike) : UnitDelay  X0=0  SampleTime=Ts
  hold values 1 : Subsystem  TreatAsAtomicUnit=on
      settings: RTWFcnNameOpts=Auto  RTWFileNameOpts=Auto
  hold values 2 : Subsystem  TreatAsAtomicUnit=on
      settings: RTWFcnNameOpts=Auto  RTWFileNameOpts=Auto
  no resetting of position : Constant  Value=0
  djerk : Outport  Port=1
  reset : Outport  Port=2
  start : Outport  Port=3
  wires:
  [td4] -> Sum6/2
  Mux2/1 -> Saturation1/1
  Sum14/1 -> Mux2/2
  Unit Delay7/1 -> Sum14/1
  Sum12/1 -> Unit Delay7/1, Sum14/2
  [td8] -> Sum12/2
  [td4] -> Sum12/1
  no resetting of position/1 -> Unit Delay9/1, Sum11/2
  Unit Delay9/1 -> Sum11/1
  Sum11/1 -> Mux2/4
  Sum15/1 -> Mux2/3
  Sum13/1 -> Mux2/1
  [td8] -> Sum15/2, Unit Delay8/1
  Unit Delay8/1 -> Sum15/1
  Unit Delay6/1 -> Sum13/1
  Sum6/1 -> Sum13/2, Unit Delay6/1
  [td8] -> Sum6/4
  [td6] -> Sum6/3
  [td2] -> Sum6/1
  Saturation1/1 -> reset/1
  Constant18/1 -> Switch16/1
  Sum3/1 -> Switch16/3
  Switch16/1 -> Unit Delay/1
  Unit Delay/1 -> [t], Sum3/2
  Constant17/1 -> Sum3/1
  Generate start/1(Out) -> Switch16/2, Saturation3/1
  [t16] -> Selector/1
  Selector/1 -> Relational Operator/1
  [t] -> Relational Operator/2
  [t16] -> Selector1/1
  Selector1/1 -> Relational Operator1/1
  [t] -> Relational Operator1/2
  [t16] -> Selector2/1
  Selector2/1 -> Relational Operator2/1
  [t] -> Relational Operator2/2
  [t16] -> Selector3/1
  Selector3/1 -> Relational Operator3/1
  [t] -> Relational Operator3/2
  [t16] -> Selector4/1
  Selector4/1 -> Relational Operator4/1
  [t] -> Relational Operator4/2
  [t16] -> Selector5/1
  Selector5/1 -> Relational Operator5/1
  [t] -> Relational Operator5/2
  [t16] -> Selector6/1
  Selector6/1 -> Relational Operator6/1
  [t] -> Relational Operator6/2
  [t16] -> Selector7/1
  Selector7/1 -> Relational Operator7/1
  [t] -> Relational Operator7/2
  [t16] -> Selector8/1
  Selector8/1 -> Relational Operator8/1
  [t] -> Relational Operator8/2
  [t16] -> Selector9/1
  Selector9/1 -> Relational Operator9/1
  [t] -> Relational Operator9/2
  [t16] -> Selector10/1
  Selector10/1 -> Relational Operator10/1
  [t] -> Relational Operator10/2
  [t16] -> Selector11/1
  Selector11/1 -> Relational Operator11/1
  [t] -> Relational Operator11/2
  [t16] -> Selector12/1
  Selector12/1 -> Relational Operator12/1
  [t] -> Relational Operator12/2
  [t16] -> Selector13/1
  Selector13/1 -> Relational Operator13/1
  [t] -> Relational Operator13/2
  [t16] -> Selector14/1
  Selector14/1 -> Relational Operator14/1
  [t] -> Relational Operator14/2
  [t16] -> Selector15/1
  Selector15/1 -> Relational Operator15/1
  [t] -> Relational Operator15/2
  Switch15/1 -> Sum/16
  [dd] -> Switch/1
  Constant1/1 -> Switch/3
  Relational Operator/1 -> Switch/2
  [dd] -> Switch1/1
  Constant2/1 -> Switch1/3
  [dd] -> Switch2/1
  Constant3/1 -> Switch2/3
  Relational Operator2/1 -> Switch2/2
  [dd] -> Switch3/1
  Constant4/1 -> Switch3/3
  [dd] -> Switch4/1
  Constant5/1 -> Switch4/3
  Relational Operator4/1 -> Switch4/2
  [dd] -> Switch5/1
  Constant6/1 -> Switch5/3
  [dd] -> Switch6/1
  Constant7/1 -> Switch6/3
  Relational Operator6/1 -> Switch6/2
  [dd] -> Switch7/1
  Constant8/1 -> Switch7/3
  [dd] -> Switch8/1
  Constant9/1 -> Switch8/3
  [dd] -> Switch9/1
  Constant10/1 -> Switch9/3
  [dd] -> Switch10/1
  Constant11/1 -> Switch10/3
  Relational Operator10/1 -> Switch10/2
  [dd] -> Switch11/1
  Constant12/1 -> Switch11/3
  [dd] -> Switch12/1
  Constant13/1 -> Switch12/3
  Relational Operator12/1 -> Switch12/2
  [dd] -> Switch13/1
  Constant14/1 -> Switch13/3
  [dd] -> Switch14/1
  Constant15/1 -> Switch14/3
  Relational Operator14/1 -> Switch14/2
  Switch/1 -> Sum/1
  Switch1/1 -> Sum/2
  Switch2/1 -> Sum/3
  Switch3/1 -> Sum/4
  Switch4/1 -> Sum/5
  Switch5/1 -> Sum/6
  Switch6/1 -> Sum/7
  Switch7/1 -> Sum/8
  Switch8/1 -> Sum/9
  Switch9/1 -> Sum/10
  Switch10/1 -> Sum/11
  Switch11/1 -> Sum/12
  Switch12/1 -> Sum/13
  Switch13/1 -> Sum/14
  Switch14/1 -> Sum/15
  Relational Operator11/1 -> Switch11/2, [td6]
  [dd] -> Switch15/1
  Constant16/1 -> Switch15/3
  Relational Operator15/1 -> Switch15/2, [td8]
  Relational Operator1/1 -> Switch1/2
  Relational Operator3/1 -> Switch3/2, [td2]
  Relational Operator5/1 -> Switch5/2
  Relational Operator7/1 -> Switch7/2, [td4]
  Relational Operator9/1 -> Switch9/2
  Relational Operator13/1 -> Switch13/2
  t,d/1 -> Demux/1
  Demux/1 -> Calculate Switching Times/1  "times"
  Calculate Switching Times/1 -> hold values 1/1(In1), Selector17/1
  Selector17/1 -> [tfinal]
  Demux/2 -> hold values 2/1(In1)
  hold values 2/1(Out1) -> [dd]
  hold values 1/1(Out1) -> [t16]
  [ready] -> Enable start/1(In)
  enable/1 -> Enable start/Enable, Logical Operator1/1
  Logical Operator/1 -> Determine  direction/Trigger
  Determine  direction/1(dir) -> [dir]
  Memory3/1 -> Logical Operator/1
  Relational Operator17/1 -> Logical Operator2/1
  [ready] -> Logical Operator2/2
  Constant19/1 -> Relational Operator17/2
  [dir] -> Relational Operator17/1
  Logical Operator1/1 -> Logical Operator2/3
  Logical Operator2/1 -> Memory3/1
  Enable start/1(Out) -> Generate start/1(In), Logical Operator/2
  Settling time/1 -> Sum2/2
  [t] -> Relational Operator16/1
  Sum2/1 -> Relational Operator16/2
  Relational Operator16/1 -> [ready]
  Memory4/1 -> [start]
  [start] -> hold values 1/Trigger
  [start] -> hold values 2/Trigger
  Saturation3/1 -> Memory4/1, start/1
  Relational Operator8/1 -> Switch8/2
  [tfinal] -> Sum2/1
  Sdir/1 -> Switch17/2
  Constant20/1 -> Switch17/3
  [dir] -> Switch17/1
  Switch17/1 -> Product1/1
  Sum/1 -> Product1/2
  Unit Delay10/1 -> djerk/1
  Product1/1 -> Unit Delay10/1
